simulink library "persistentExcitation_ul"  (R2018a)
settings: Solver=VariableStepAuto  StartTime=0.0  StopTime=10.0  RelTol=1e-3
undefined symbols (not defined in the file): ctrl
settings Model: Creator=mitch  LastModifiedBy=M.Cobb

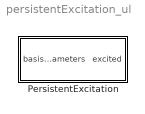
== system persistentExcitation_ul ==
  PersistentExcitation : Subsystem

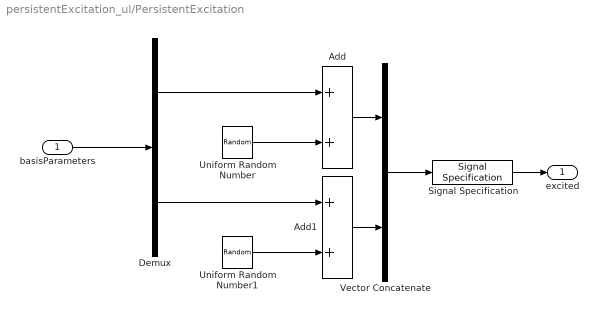
== system persistentExcitation_ul/PersistentExcitation ==
  basisParameters : Inport  PortDimensions=[1 2]
  Add : Sum
  Add1 : Sum
  Demux : Demux  Outputs=2
  Signal Specification : SignalSpecification  Dimensions=[1 2]
  Uniform Random Number : UniformRandomNumber  Minimum=-ctrl.persistenExcitationAzimuth_norm  Maximum=ctrl.persistenExcitationAzimuth_norm
  Uniform Random Number1 : UniformRandomNumber  Minimum=-ctrl.persistenExcitationZenith_norm  Maximum=ctrl.persistenExcitationZenith_norm
  Vector Concatenate : Concatenate
  excited : Outport  PortDimensions=[1 2]
  wires:
  Signal Specification/1 -> excited/1
  basisParameters/1 -> Demux/1
  Vector Concatenate/1 -> Signal Specification/1
  Add/1 -> Vector Concatenate/1
  Add1/1 -> Vector Concatenate/2
  Demux/1 -> Add/1
  Demux/2 -> Add1/1
  Uniform Random Number/1 -> Add/2
  Uniform Random Number1/1 -> Add1/2
